simulink model "HevIpsPowertrainController"  (R2023b)
settings: configuration reference "VehicleFixed10ms" (kept outside this file)
undefined symbols (not defined in the file): CtrlBcuTrlrBrkGain, CtrlVcuHevIpsBattChrgPwrMax, CtrlVcuHevIpsBattDischrgPwrMax, CtrlVcuHevIpsChrgLmtBpt, CtrlVcuHevIpsDischrgLmtBpt, CtrlVcuHevIpsEngPwr, CtrlVcuHevIpsEngSpd, CtrlVcuHevIpsEngTrq, CtrlVcuHevIpsEngTrqWhl, CtrlVcuHevIpsEVSpdLmt, CtrlVcuHevIpsGenPwrMax, CtrlVcuHevIpsGenTrqMax, CtrlVcuHevIpsMotPwr, CtrlVcuHevIpsN_idle, CtrlVcuHevIpsNsysWhl, CtrlVcuHevIpsRegenBrkCutOff, CtrlVcuHevIpsRegenBrkSpdBpt, CtrlVcuHevIpsSocBpt, CtrlVcuHevIpsSOCChrgFactor, CtrlVcuHevIpsSOCmin, CtrlVcuHevIpsSOCtarget, CtrlVcuHevIpsSysTrqWhl, PlntBrkActrBoreFrnt, PlntBrkFrntBias, PlntBrkKinFricCffFrnt, PlntBrkNumPadsFrnt, PlntBrkPadMeanRadiusFrnt, PlntBrkPrsFctr, PlntBrkRearBias, PlntDiffrntlRatio, PlntEM1EffTbl, PlntEM1Spd, PlntEM1Trq, PlntEM1TrqEff, PlntEM2EffTbl, PlntEM2Spd, PlntEM2Trq, PlntEM2TrqEff, PlntHevIpsP1SunRingRatio, PlntHevIpsP2GearRatio
libraries: simulink x19, autolibutils x4, slpidlib x1
(part 1 of 2)
settings Model: DataDictionary=VirtualVehicleTemplate.sldd  ModifiedByFormat=The MathWorks, Inc.  Creator=The MathWorks, Inc.  LastModifiedBy=The MathWorks, Inc.
settings ConfigSetRef: SourceName=VehicleFixed10ms

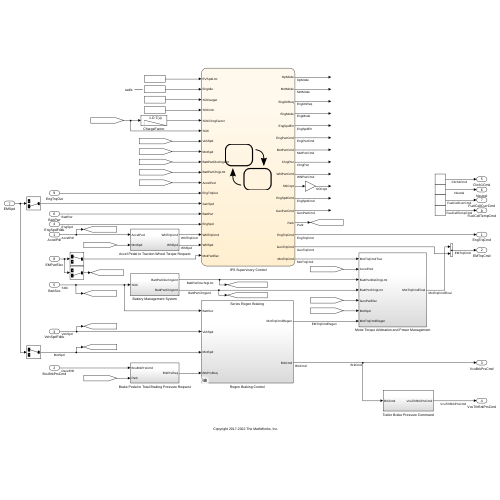
[thumbnail: Simulink's stored preview of the top-level diagram]
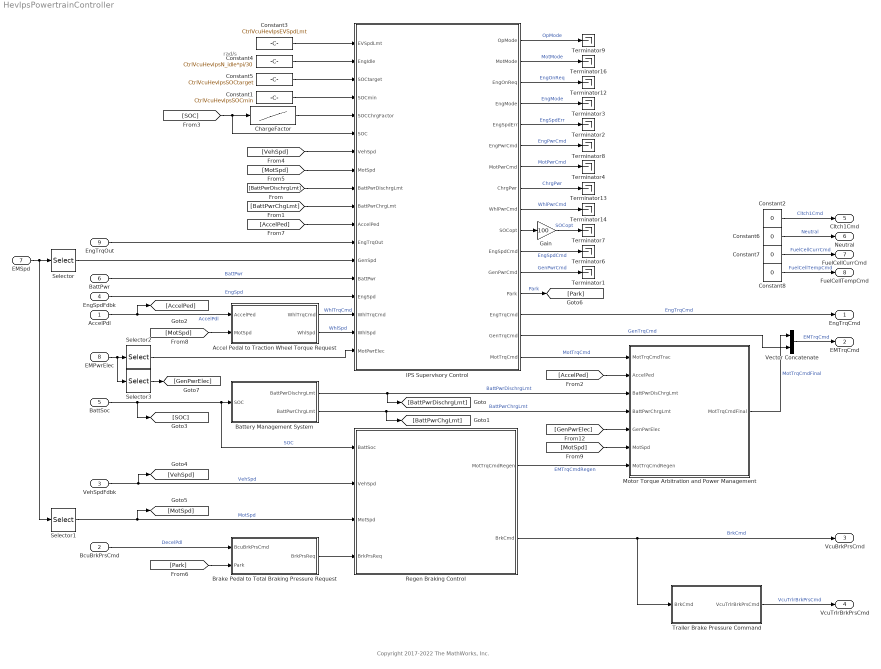
== system HevIpsPowertrainController ==
  note: rad/s
  note: Copyright 2017-2022 The MathWorks, Inc.
  AccelPdl : Inport  OutDataTypeStr=double  PortDimensions=1
  BcuBrkPrsCmd : Inport  Port=2  OutDataTypeStr=double  PortDimensions=4
  VehSpdFdbk : Inport  Port=3  OutDataTypeStr=double  PortDimensions=1
  EngSpdFdbk : Inport  Port=4  OutDataTypeStr=double  PortDimensions=1
  BattSoc : Inport  Port=5  OutDataTypeStr=double  PortDimensions=1
  BattPwr : Inport  Port=6  OutDataTypeStr=double  PortDimensions=1
  EMSpd : Inport  Port=7  OutDataTypeStr=double  PortDimensions=2
  EMPwrElec : Inport  Port=8  OutDataTypeStr=double  PortDimensions=2
  EngTrqOut : Inport  Port=9  OutDataTypeStr=double  PortDimensions=1
  Accel Pedal to Traction Wheel Torque Request : Subsystem  InitFcn=[~]=autosharedicon('autolibinternalvvblock',gcb,0);
  Battery Management System : Subsystem
  Brake Pedal to Total Braking Pressure Request : Subsystem
  ChargeFactor : Lookup_n-D  NumberOfTableDimensions=1  BreakpointsForDimension1=[20 80]  Table=CtrlVcuHevIpsSOCChrgFactor  ExtrapMethod=Clip  UseLastTableValue=on  InternalRulePriority=Speed  RndMeth=Simplest
  Constant1 : Constant  Value=CtrlVcuHevIpsSOCmin  SampleTime=-1
  Constant{2,6..8} (4 alike) : Constant  Value=0  SampleTime=-1
  Constant3 : Constant  Value=CtrlVcuHevIpsEVSpdLmt  SampleTime=-1
  Constant4 : Constant  Value=CtrlVcuHevIpsN_idle*pi/30  SampleTime=-1
  Constant5 : Constant  Value=CtrlVcuHevIpsSOCtarget  SampleTime=-1
  Gain : Gain  Gain=100
  IPS Supervisory Control : Stateflow chart  TreatAsAtomicUnit=on
  Motor Torque Arbitration and Power Management : Subsystem
  Regen Braking Control : Subsystem  Variant=on  VariantControlMode=label  VariantControl=(default)  LabelModeActiveChoice=Variant
  Selector : Selector  InputPortWidth=2  IndexOptions=Index vector (dialog)  Indices=[2]  OutputSizes=1
  Selector1 : Selector  InputPortWidth=2  IndexOptions=Index vector (dialog)  Indices=[1]  OutputSizes=1
  Selector2 : Selector  InputPortWidth=2  IndexOptions=Index vector (dialog)  Indices=[1]  OutputSizes=1
  Selector3 : Selector  InputPortWidth=2  IndexOptions=Index vector (dialog)  Indices=[2]  OutputSizes=1
  Terminator{1..4,6..9,12..14,16} (12 alike) : Terminator
  Trailer Brake Pressure Command : Subsystem
  Vector Concatenate : Concatenate
  EngTrqCmd : Outport  OutDataTypeStr=double  PortDimensions=1  VectorParamsAs1DForOutWhenUnconnected=off
  EMTrqCmd : Outport  Port=2  OutDataTypeStr=double  PortDimensions=2  VectorParamsAs1DForOutWhenUnconnected=off
  VcuBrkPrsCmd : Outport  Port=3  OutDataTypeStr=double  PortDimensions=4  VectorParamsAs1DForOutWhenUnconnected=off
  VcuTrlrBrkPrsCmd : Outport  Port=4  PortDimensions=6  VectorParamsAs1DForOutWhenUnconnected=off
  Cltch1Cmd : Outport  Port=5  OutDataTypeStr=double  PortDimensions=1  VectorParamsAs1DForOutWhenUnconnected=off
  Neutral : Outport  Port=6  OutDataTypeStr=double  PortDimensions=1  VectorParamsAs1DForOutWhenUnconnected=off
  FuelCellCurrCmd : Outport  Port=7  OutDataTypeStr=double  PortDimensions=1
  FuelCellTempCmd : Outport  Port=8  OutDataTypeStr=double  PortDimensions=1
  wires:
  AccelPdl/1 -> Accel Pedal to Traction Wheel Torque Request/1(AccelPed), [AccelPed]  "AccelPdl"
  BcuBrkPrsCmd/1 -> Brake Pedal to Total Braking Pressure Request/1(BcuBrkPrsCmd)  "DecelPdl"
  VehSpdFdbk/1 -> [VehSpd], Regen Braking Control/2("VehSpd ")  "VehSpd"
  EngSpdFdbk/1 -> IPS Supervisory Control/15(EngSpd)  "EngSpd"
  BattPwr/1 -> IPS Supervisory Control/14(BattPwr)  "BattPwr"
  BattSoc/1 -> [SOC], Regen Braking Control/1("BattSoc "), Battery Management System/1(SOC)  "SOC"
  Selector1/1 -> [MotSpd], Regen Braking Control/3("MotSpd ")  "MotSpd"
  Battery Management System/2(BattPwrChrgLmt) -> [BattPwrChgLmt], Motor Torque Arbitration and Power Management/4("BattPwrChrgLmt ")  "BattPwrChrgLmt"
  Battery Management System/1(BattPwrDischrgLmt) -> Motor Torque Arbitration and Power Management/3(BattPwrDisChrgLmt), [BattPwrDischrgLmt]  "BattPwrDischrgLmt"
  IPS Supervisory Control/1(OpMode) -> Terminator9/1  "OpMode"
  IPS Supervisory Control/6(EngPwrCmd) -> Terminator8/1  "EngPwrCmd"
  IPS Supervisory Control/3(EngOnReq) -> Terminator12/1  "EngOnReq"
  IPS Supervisory Control/7(MotPwrCmd) -> Terminator4/1  "MotPwrCmd"
  [SOC] -> IPS Supervisory Control/6(SOC), ChargeFactor/1
  [VehSpd] -> IPS Supervisory Control/7(VehSpd)
  Constant3/1 -> IPS Supervisory Control/1(EVSpdLmt)
  [BattPwrDischrgLmt] -> IPS Supervisory Control/9(BattPwrDischrgLmt)
  [BattPwrChgLmt] -> IPS Supervisory Control/10(BattPwrChrgLmt)
  Accel Pedal to Traction Wheel Torque Request/1(WhlTrqCmd) -> IPS Supervisory Control/16(WhlTrqCmd)  "WhlTrqCmd"
  Constant4/1 -> IPS Supervisory Control/2(EngIdle)
  Accel Pedal to Traction Wheel Torque Request/2(WhlSpd) -> IPS Supervisory Control/17(WhlSpd)  "WhlSpd"
  IPS Supervisory Control/16(MotTrqCmd) -> Motor Torque Arbitration and Power Management/1(MotTrqCmdTrac)  "MotTrqCmd"
  Brake Pedal to Total Braking Pressure Request/1(BrkPrsReq) -> Regen Braking Control/4("BrkPrsReq ")
  Regen Braking Control/1(" MotTrqCmdRegen") -> Motor Torque Arbitration and Power Management/7(MotTrqCmdRegen)  "EMTrqCmdRegen"
  IPS Supervisory Control/10(SOCopt) -> Gain/1
  IPS Supervisory Control/8(ChrgPwr) -> Terminator13/1  "ChrgPwr"
  IPS Supervisory Control/9(WhlPwrCmd) -> Terminator14/1  "WhlPwrCmd"
  [MotSpd] -> IPS Supervisory Control/8(MotSpd)
  Gain/1 -> Terminator7/1  "SOCopt"
  IPS Supervisory Control/4(EngMode) -> Terminator3/1  "EngMode"
  IPS Supervisory Control/11(EngSpdCmd) -> Terminator6/1  "EngSpdCmd"
  IPS Supervisory Control/2(MotMode) -> Terminator16/1  "MotMode"
  Constant5/1 -> IPS Supervisory Control/3(SOCtarget)
  ChargeFactor/1 -> IPS Supervisory Control/5(SOCChrgFactor)
  [AccelPed] -> IPS Supervisory Control/11(AccelPed)
  IPS Supervisory Control/5(EngSpdErr) -> Terminator2/1  "EngSpdErr"
  [MotSpd] -> Accel Pedal to Traction Wheel Torque Request/2(MotSpd)
  [AccelPed] -> Motor Torque Arbitration and Power Management/2(AccelPed)
  Selector/1 -> IPS Supervisory Control/13(GenSpd)
  Selector3/1 -> [GenPwrElec]
  IPS Supervisory Control/12(GenPwrCmd) -> Terminator1/1  "GenPwrCmd"
  EMPwrElec/1 -> Selector3/1, Selector2/1
  Motor Torque Arbitration and Power Management/1(MotTrqCmdFinal) -> Vector Concatenate/1  "MotTrqCmdFinal"
  Constant1/1 -> IPS Supervisory Control/4(SOCmin)
  IPS Supervisory Control/15(GenTrqCmd) -> Vector Concatenate/2  "GenTrqCmd"
  IPS Supervisory Control/14(EngTrqCmd) -> EngTrqCmd/1  "EngTrqCmd"
  EngTrqOut/1 -> IPS Supervisory Control/12(EngTrqOut)
  IPS Supervisory Control/13(Park) -> [Park]  "Park"
  [Park] -> Brake Pedal to Total Braking Pressure Request/2(Park)
  [MotSpd] -> Motor Torque Arbitration and Power Management/6(MotSpd)
  [GenPwrElec] -> Motor Torque Arbitration and Power Management/5(GenPwrElec)
  Vector Concatenate/1 -> EMTrqCmd/1  "EMTrqCmd"
  EMSpd/1 -> Selector1/1, Selector/1
  Constant6/1 -> Neutral/1  "Neutral"
  Constant2/1 -> Cltch1Cmd/1  "Cltch1Cmd"
  Selector2/1 -> IPS Supervisory Control/18(MotPwrElec)
  Constant7/1 -> FuelCellCurrCmd/1  "FuelCellCurrCmd"
  Constant8/1 -> FuelCellTempCmd/1  "FuelCellTempCmd"
  Regen Braking Control/2(" BrkCmd") -> Trailer Brake Pressure Command/1(BrkCmd), VcuBrkPrsCmd/1  "BrkCmd"
  Trailer Brake Pressure Command/1(VcuTrlrBrkPrsCmd) -> VcuTrlrBrkPrsCmd/1  "VcuTrlrBrkPrsCmd"

== system HevIpsPowertrainController/Accel Pedal to Traction Wheel Torque Request ==
  AccelPed : Inport
  MotSpd : Inport  Port=2
  MaxSysTrqWhlVsWhlSpd : Lookup_n-D  NumberOfTableDimensions=1  BreakpointsForDimension1=CtrlVcuHevIpsNsysWhl  Table=CtrlVcuHevIpsSysTrqWhl  ExtrapMethod=Clip  UseLastTableValue=on  InternalRulePriority=Speed  OutDataTypeStr=Inherit: Inherit from 'Table data'  RndMeth=Simplest
  MotSpdToWhlSpd : Gain  Gain=1/(PlntHevIpsP2GearRatio)/PlntDiffrntlRatio
  Product1 : Product
  rads_to_rpm : Gain  Gain=30/pi
  WhlTrqCmd : Outport  VectorParamsAs1DForOutWhenUnconnected=off
  WhlSpd : Outport  Port=2  VectorParamsAs1DForOutWhenUnconnected=off
  wires:
  rads_to_rpm/1 -> MaxSysTrqWhlVsWhlSpd/1
  MotSpdToWhlSpd/1 -> rads_to_rpm/1, WhlSpd/1
  Product1/1 -> WhlTrqCmd/1
  MotSpd/1 -> MotSpdToWhlSpd/1
  MaxSysTrqWhlVsWhlSpd/1 -> Product1/2
  AccelPed/1 -> Product1/1

== system HevIpsPowertrainController/Battery Management System ==
  note: Limit battery charge / discharge power based on SOC
  SOC : Inport
  ChrgLmt : Lookup_n-D  NumberOfTableDimensions=1  BreakpointsForDimension1=CtrlVcuHevIpsSocBpt  Table=CtrlVcuHevIpsChrgLmtBpt  ExtrapMethod=Clip  UseLastTableValue=on  InternalRulePriority=Speed  RndMeth=Simplest
  DischrgLmt : Lookup_n-D  NumberOfTableDimensions=1  BreakpointsForDimension1=CtrlVcuHevIpsSocBpt  Table=CtrlVcuHevIpsDischrgLmtBpt  ExtrapMethod=Clip  UseLastTableValue=on  InternalRulePriority=Speed  RndMeth=Simplest
  MaxChrg : Constant  Value=CtrlVcuHevIpsBattChrgPwrMax  SampleTime=-1
  MaxDischrg : Constant  Value=CtrlVcuHevIpsBattDischrgPwrMax  SampleTime=-1
  Product : Product
  Product1 : Product
  BattPwrDischrgLmt : Outport  VectorParamsAs1DForOutWhenUnconnected=off
  BattPwrChrgLmt : Outport  Port=2  VectorParamsAs1DForOutWhenUnconnected=off
  wires:
  SOC/1 -> DischrgLmt/1, ChrgLmt/1
  MaxChrg/1 -> Product1/2
  MaxDischrg/1 -> Product/2
  Product/1 -> BattPwrDischrgLmt/1
  Product1/1 -> BattPwrChrgLmt/1
  ChrgLmt/1 -> Product1/1
  DischrgLmt/1 -> Product/1

== system HevIpsPowertrainController/Brake Pedal to Total Braking Pressure Request ==
  BcuBrkPrsCmd : Inport
  Park : Inport  Port=2
  Front Bias : Constant  Value=PlntBrkFrntBias
  Gain4 : Gain  Gain=PlntBrkPrsFctr
  Mux : Mux
  Product : Product
  Rear Bias : Constant  Value=PlntBrkRearBias
  Terminator : Terminator
  BrkPrsReq : Outport  VectorParamsAs1DForOutWhenUnconnected=off
  wires:
  BcuBrkPrsCmd/1 -> Product/2
  Mux/1 -> Product/1
  Rear Bias/1 -> Mux/4, Mux/3
  Front Bias/1 -> Mux/1, Mux/2
  Gain4/1 -> BrkPrsReq/1
  Product/1 -> Gain4/1
  Park/1 -> Terminator/1

== system HevIpsPowertrainController/IPS Supervisory Control/Engine_Control.Run.TrqCalc ==
  EngPwrCmd : Inport
  f : TriggerPort  TriggerType=function-call  VariantControl=Variant  StatesWhenEnabling=reset
      settings: CopyFcn=Stateflow.SLINSF.SimulinkMan.removeBlockPreDeleteFcn  PreDeleteFcn=Stateflow.SLINSF.SimulinkMan.unsafePredeleteFcn
  OptimalEngineSpeed : Lookup_n-D  NumberOfTableDimensions=1  BreakpointsForDimension1=[0 CtrlVcuHevIpsEngPwr(1,1:15)]  Table=[CtrlVcuHevIpsN_idle CtrlVcuHevIpsEngSpd(1,1:15)]  ExtrapMethod=Clip  UseLastTableValue=on  InternalRulePriority=Speed  RndMeth=Simplest
  OptimalEngineTorque : Lookup_n-D  NumberOfTableDimensions=1  BreakpointsForDimension1=[0 CtrlVcuHevIpsEngPwr(1,1:15)]  Table=[0 CtrlVcuHevIpsEngTrq(1,1:15)]  ExtrapMethod=Clip  UseLastTableValue=on  InternalRulePriority=Speed  RndMeth=Simplest
  rpm_to_rads : Gain  Gain=pi/30
  EngTrqCmd : Outport  VectorParamsAs1DForOutWhenUnconnected=off
  EngSpdCmd : Outport  Port=2  VectorParamsAs1DForOutWhenUnconnected=off
  wires:
  rpm_to_rads/1 -> EngSpdCmd/1
  OptimalEngineSpeed/1 -> rpm_to_rads/1
  EngPwrCmd/1 -> OptimalEngineTorque/1, OptimalEngineSpeed/1
  OptimalEngineTorque/1 -> EngTrqCmd/1

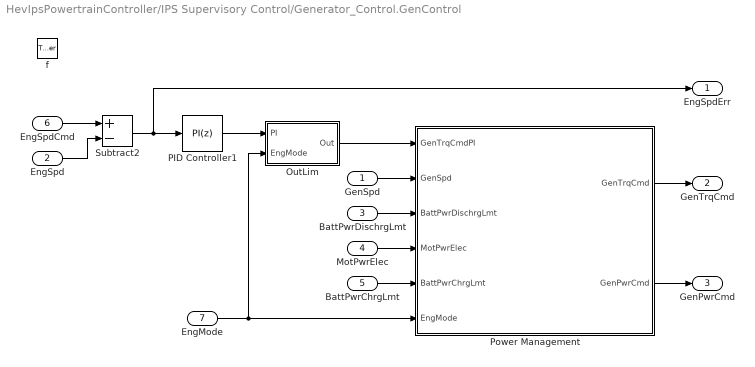
== system HevIpsPowertrainController/IPS Supervisory Control/Generator_Control.GenControl ==
  GenSpd : Inport
  EngSpd : Inport  Port=2
  BattPwrDischrgLmt : Inport  Port=3
  MotPwrElec : Inport  Port=4
  BattPwrChrgLmt : Inport  Port=5
  EngSpdCmd : Inport  Port=6
  EngMode : Inport  Port=7
  f : TriggerPort  TriggerType=function-call  VariantControl=Variant  StatesWhenEnabling=reset  SampleTime=-1
      settings: CopyFcn=Stateflow.SLINSF.SimulinkMan.removeBlockPreDeleteFcn  PreDeleteFcn=Stateflow.SLINSF.SimulinkMan.unsafePredeleteFcn
  OutLim : Subsystem
  PID Controller1 : slpidlib/PID Controller  Controller=PI  Form=Parallel  TimeDomain=Discrete-time  UseExternalTs=off  SampleTime=-1  IntegratorMethod=Forward Euler  FilterMethod=Forward Euler  ControllerParametersSource=internal  P=1  I=0.5  UseKiTs=off  D=1  N=100  UseFilter=on  TunerSelectOption=Transfer Function Based (PID Tuner App)  ZeroCross=off  InitialConditionSource=internal  InitialConditionForIntegrator=0  InitialConditionForFilter=0  DifferentiatorICPrevScaledInput=0  ExternalReset=none  TrackingMode=off  Kt=1  LimitOutput=on  SatLimitsSource=internal  UpperSaturationLimit=CtrlVcuHevIpsGenTrqMax  LowerSaturationLimit=-CtrlVcuHevIpsGenTrqMax  LinearizeAsGain=on  AntiWindupMode=clamping  Kb=1  LimitIntegrator=off  UpperIntegratorSaturationLimit=inf  LowerIntegratorSaturationLimit=-inf  POutMin=[]  POutMax=[]  IOutMin=[]  IOutMax=[]  DOutMin=[]  DOutMax=[]  NOutMin=[]  NOutMax=[]  SumOutMin=[]  SumOutMax=[]  SaturationOutMin=[]  SaturationOutMax=[]  PParamMin=[]  PParamMax=[]  IParamMin=[]  IParamMax=[]  DParamMin=[]  DParamMax=[]  NParamMin=[]  NParamMax=[]  KbParamMin=[]  KbParamMax=[]  KtParamMin=[]  KtParamMax=[]  KbOutMin=[]  KbOutMax=[]  KtOutMin=[]  KtOutMax=[]  IntegratorOutMin=[]  IntegratorOutMax=[]  FilterOutMin=[]  FilterOutMax=[]  SumI1OutMin=[]  SumI1OutMax=[]  SumI2OutMin=[]  SumI2OutMax=[]  SumI3OutMin=[]  SumI3OutMax=[]  SumI4OutMin=[]  SumI4OutMax=[]  SumDOutMin=[]  SumDOutMax=[]  DifferentiatorOutMin=[]  DifferentiatorOutMax=[]  FilterDiffOutCoefMin=[]  FilterDiffOutCoefMax=[]  ReciprocalOutMin=[]  ReciprocalOutMax=[]  SumDenOutMin=[]  SumDenOutMax=[]  SumNumOutMin=[]  SumNumOutMax=[]  DivideOutMin=[]  DivideOutMax=[]  UdiffTsProdOutMin=[]  UdiffTsProdOutMax=[]  NTsProdOutMin=[]  NTsProdOutMax=[]  UintegralTsProdOutMin=[]  UintegralTsProdOutMax=[]  UngainTsProdOutMin=[]  UngainTsProdOutMax=[]  ClampingZeroOutDataTypeStr=Inherit: Inherit via back propagation  ClampingZeroOutMin=[]  ClampingZeroOutMax=[]  FilterDenConstantOutDataTypeStr=Inherit: Inherit via back propagation  FilterDenConstantOutMin=[]  FilterDenConstantOutMax=[]  PCopyOutDataTypeStr=Inherit: Inherit via back propagation  PCopyOutMin=[]  PCopyOutMax=[]  NCopyOutDataTypeStr=Inherit: Inherit via back propagation  NCopyOutMin=[]  NCopyOutMax=[]  IntegratorContinuousStateAttributes=''  IntegratorStateMustResolveToSignalObject=off  IntegratorRTWStateStorageClass=Auto  FilterContinuousStateAttributes=''  FilterStateMustResolveToSignalObject=off  FilterRTWStateStorageClass=Auto  ParallelPVariant=InternalParameters  IdealPVariant=Disabled  IVariant=InternalParameters  DVariant=Disabled  IntegratorVariant=Discrete  SatVariant=Enabled  AWVariant=DiscClampingParallel  PCopyVariant=Disabled  TRVariant=Disabled  FdbkBlocksVariant=Forward  IdealPFdbkVariant=Disabled  SatFdbkVariant=Disabled  DerivativeFilterVariant=Disabled  NVariant=Disabled  NCopyVariant=Disabled_SignalSpec  FilterICVariant=Disabled  IntegratorICVariant=InternalICs  ExternalResetVariant=Disabled  TRSumVariant=Passthrough  SumFdbkVariant=Disabled  SumVariant=Sum_PI  TsampFilterVariant=InternalTs  TsampNgainVariant=Passthrough  TsampIntegralVariant=Disabled_SignalSpec  ExternalSaturationOutDataTypeStr=Inherit: Same as second input
  Power Management : Subsystem
  Subtract2 : Sum  Inputs=+-
  EngSpdErr : Outport  VectorParamsAs1DForOutWhenUnconnected=off
  GenTrqCmd : Outport  Port=2  VectorParamsAs1DForOutWhenUnconnected=off
  GenPwrCmd : Outport  Port=3  VectorParamsAs1DForOutWhenUnconnected=off
  wires:
  Subtract2/1 -> PID Controller1/1, EngSpdErr/1
  EngSpd/1 -> Subtract2/2
  MotPwrElec/1 -> Power Management/4(MotPwrElec)
  BattPwrDischrgLmt/1 -> Power Management/3(BattPwrDischrgLmt)
  BattPwrChrgLmt/1 -> Power Management/5(BattPwrChrgLmt)
  GenSpd/1 -> Power Management/2(GenSpd)
  EngSpdCmd/1 -> Subtract2/1
  EngMode/1 -> OutLim/2(EngMode), Power Management/6(EngMode)
  Power Management/1(GenTrqCmd) -> GenTrqCmd/1
  Power Management/2(GenPwrCmd) -> GenPwrCmd/1
  PID Controller1/1 -> OutLim/1(PI)
  OutLim/1(Out) -> Power Management/1(GenTrqCmdPI)

== system HevIpsPowertrainController/IPS Supervisory Control/Motor_Control.Mot_EV.MotTrqEV ==
  WhlTrqCmd : Inport
  f : TriggerPort  TriggerType=function-call  VariantControl=Variant  StatesWhenEnabling=reset
      settings: CopyFcn=Stateflow.SLINSF.SimulinkMan.removeBlockPreDeleteFcn  PreDeleteFcn=Stateflow.SLINSF.SimulinkMan.unsafePredeleteFcn
  WhlTrqReflectedMotTrq : Gain  Gain=1/(PlntHevIpsP2GearRatio)/PlntDiffrntlRatio
  MotTrqCmd : Outport  VectorParamsAs1DForOutWhenUnconnected=off
  wires:
  WhlTrqCmd/1 -> WhlTrqReflectedMotTrq/1
  WhlTrqReflectedMotTrq/1 -> MotTrqCmd/1

== system HevIpsPowertrainController/IPS Supervisory Control/Motor_Control.Mot_HEV.MotTrqHEV ==
  MotPwrCmd : Inport
  MotSpd : Inport  Port=2
  f : TriggerPort  TriggerType=function-call  VariantControl=Variant  StatesWhenEnabling=reset
      settings: CopyFcn=Stateflow.SLINSF.SimulinkMan.removeBlockPreDeleteFcn  PreDeleteFcn=Stateflow.SLINSF.SimulinkMan.unsafePredeleteFcn
  Elec_to_MechPwr1 : Product  Inputs=*/
  div0protect - poly1 : autolibutils/div0protect - poly  thresh=2  ZeroCross1=off  aMode=aMode
  MotTrqCmd : Outport  VectorParamsAs1DForOutWhenUnconnected=off
  wires:
  MotPwrCmd/1 -> Elec_to_MechPwr1/1
  MotSpd/1 -> div0protect - poly1/1
  div0protect - poly1/1 -> Elec_to_MechPwr1/2
  Elec_to_MechPwr1/1 -> MotTrqCmd/1

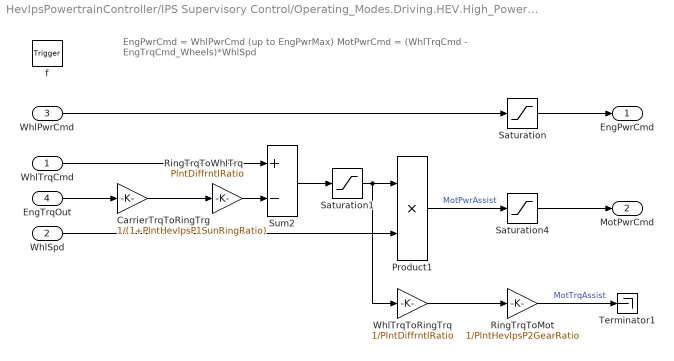
== system HevIpsPowertrainController/IPS Supervisory Control/Operating_Modes.Driving.HEV.High_Power_Charge_Deplete.OpMode4 ==
  note: EngPwrCmd = WhlPwrCmd (up to EngPwrMax)
      | MotPwrCmd =  (WhlTrqCmd - EngTrqCmd_Wheels)*WhlSpd
  WhlTrqCmd : Inport
  WhlSpd : Inport  Port=2
  WhlPwrCmd : Inport  Port=3
  EngTrqOut : Inport  Port=4
  f : TriggerPort  TriggerType=function-call  VariantControl=Variant  StatesWhenEnabling=reset
      settings: CopyFcn=Stateflow.SLINSF.SimulinkMan.removeBlockPreDeleteFcn  PreDeleteFcn=Stateflow.SLINSF.SimulinkMan.unsafePredeleteFcn
  CarrierTrqToRingTrg : Gain  Gain=1/(1+PlntHevIpsP1SunRingRatio)
  Product1 : Product
  RingTrqToMot : Gain  Gain=1/PlntHevIpsP2GearRatio
  RingTrqToWhlTrq : Gain  Gain=PlntDiffrntlRatio
  Saturation : Saturate  UpperLimit=max(CtrlVcuHevIpsEngPwr(1,1:15))  LowerLimit=0
  Saturation1 : Saturate  UpperLimit=inf  LowerLimit=0
  Saturation4 : Saturate  UpperLimit=max(CtrlVcuHevIpsMotPwr)  LowerLimit=0
  Sum2 : Sum  Inputs=+-
  Terminator1 : Terminator
  WhlTrqToRingTrq : Gain  Gain=1/PlntDiffrntlRatio
  EngPwrCmd : Outport  VectorParamsAs1DForOutWhenUnconnected=off
  MotPwrCmd : Outport  Port=2  VectorParamsAs1DForOutWhenUnconnected=off
  wires:
  CarrierTrqToRingTrg/1 -> RingTrqToWhlTrq/1
  WhlSpd/1 -> Product1/2
  WhlTrqCmd/1 -> Sum2/1
  RingTrqToWhlTrq/1 -> Sum2/2
  Sum2/1 -> Saturation1/1
  Saturation1/1 -> WhlTrqToRingTrq/1, Product1/1
  WhlTrqToRingTrq/1 -> RingTrqToMot/1
  RingTrqToMot/1 -> Terminator1/1  "MotTrqAssist"
  Product1/1 -> Saturation4/1  "MotPwrAssist"
  EngTrqOut/1 -> CarrierTrqToRingTrg/1
  Saturation/1 -> EngPwrCmd/1
  WhlPwrCmd/1 -> Saturation/1
  Saturation4/1 -> MotPwrCmd/1

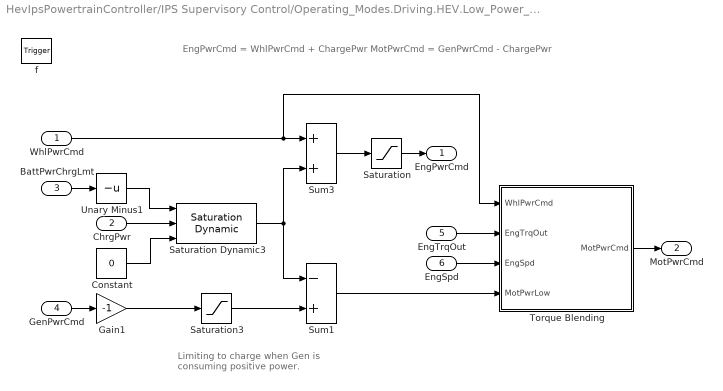
== system HevIpsPowertrainController/IPS Supervisory Control/Operating_Modes.Driving.HEV.Low_Power_Charge_Sustain.OpMode3 ==
  note: Limiting to charge when Gen
      | is consuming positive power.
  note: EngPwrCmd = WhlPwrCmd + ChargePwr
      | MotPwrCmd = GenPwrCmd - ChargePwr
  WhlPwrCmd : Inport
  ChrgPwr : Inport  Port=2
  BattPwrChrgLmt : Inport  Port=3
  GenPwrCmd : Inport  Port=4
  EngTrqOut : Inport  Port=5
  EngSpd : Inport  Port=6
  f : TriggerPort  TriggerType=function-call  VariantControl=Variant  StatesWhenEnabling=reset
      settings: CopyFcn=Stateflow.SLINSF.SimulinkMan.removeBlockPreDeleteFcn  PreDeleteFcn=Stateflow.SLINSF.SimulinkMan.unsafePredeleteFcn
  Constant : Constant  Value=0
  Gain1 : Gain  Gain=-1
  Saturation : Saturate  UpperLimit=max(CtrlVcuHevIpsEngPwr(1,1:15))  LowerLimit=0
  Saturation Dynamic3 : simulink/Discontinuities/Saturation Dynamic  OutMin=[]  OutMax=[]  OutDataTypeStr=Inherit: Same as second input  OutDataType=fixdt(1, 16)  OutScaling=2^-10  DoSatur=off
  Saturation3 : Saturate  UpperLimit=0  LowerLimit=-CtrlVcuHevIpsGenPwrMax
  Sum1 : Sum  Inputs=-+
  Sum3 : Sum
  Torque Blending : Subsystem
  Unary Minus1 : UnaryMinus
  EngPwrCmd : Outport  VectorParamsAs1DForOutWhenUnconnected=off
  MotPwrCmd : Outport  Port=2  VectorParamsAs1DForOutWhenUnconnected=off
  wires:
  Unary Minus1/1 -> Saturation Dynamic3/1
  Sum3/1 -> Saturation/1
  ChrgPwr/1 -> Saturation Dynamic3/2
  Saturation/1 -> EngPwrCmd/1
  Saturation Dynamic3/1 -> Sum1/1, Sum3/2
  GenPwrCmd/1 -> Gain1/1
  Gain1/1 -> Saturation3/1
  BattPwrChrgLmt/1 -> Unary Minus1/1
  Constant/1 -> Saturation Dynamic3/3
  WhlPwrCmd/1 -> Sum3/1, Torque Blending/1(WhlPwrCmd)
  Saturation3/1 -> Sum1/2
  EngTrqOut/1 -> Torque Blending/2(EngTrqOut)
  EngSpd/1 -> Torque Blending/3(EngSpd)
  Sum1/1 -> Torque Blending/4(MotPwrLow)
  Torque Blending/1(MotPwrCmd) -> MotPwrCmd/1

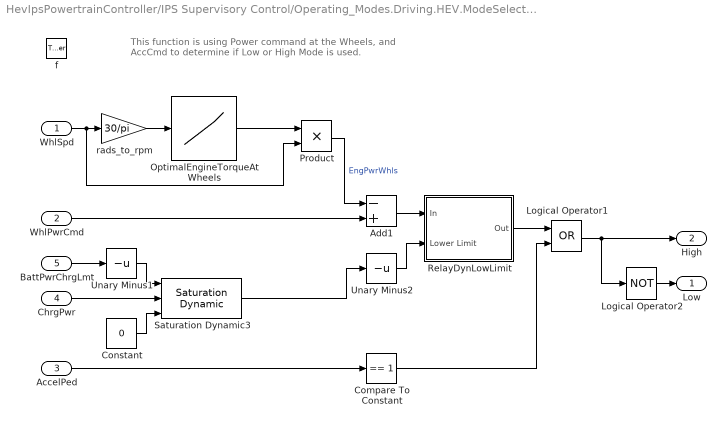
== system HevIpsPowertrainController/IPS Supervisory Control/Operating_Modes.Driving.HEV.ModeSelection ==
  note: This function is using Power command at the Wheels,
      | and AccCmd to determine if Low or High Mode is used.
  WhlSpd : Inport  PortDimensions=1
  WhlPwrCmd : Inport  Port=2  PortDimensions=1
  AccelPed : Inport  Port=3  PortDimensions=1
  ChrgPwr : Inport  Port=4
  BattPwrChrgLmt : Inport  Port=5
  f : TriggerPort  TriggerType=function-call  VariantControl=Variant  StatesWhenEnabling=reset
      settings: CopyFcn=Stateflow.SLINSF.SimulinkMan.removeBlockPreDeleteFcn  PreDeleteFcn=Stateflow.SLINSF.SimulinkMan.unsafePredeleteFcn
  Add1 : Sum  Inputs=-+
  Compare To Constant : simulink/Logic and Bit Operations/Compare To Constant  relop===  const=1  OutDataTypeStr=boolean
  Constant : Constant  Value=0
  Logical Operator1 : Logic  Operator=OR  AllPortsSameDT=off  OutDataTypeStr=boolean
  Logical Operator2 : Logic  Operator=NOT  AllPortsSameDT=off  OutDataTypeStr=boolean
  OptimalEngineTorqueAtWheels : Lookup_n-D  NumberOfTableDimensions=1  BreakpointsForDimension1=CtrlVcuHevIpsNsysWhl  Table=CtrlVcuHevIpsEngTrqWhl  ExtrapMethod=Clip  UseLastTableValue=on  InternalRulePriority=Speed  RndMeth=Simplest
  Product : Product
  RelayDynLowLimit : Subsystem
  Saturation Dynamic3 : simulink/Discontinuities/Saturation Dynamic  OutMin=[]  OutMax=[]  OutDataTypeStr=Inherit: Same as second input  OutDataType=fixdt(1, 16)  OutScaling=2^-10  DoSatur=off
  Unary Minus1 : UnaryMinus
  Unary Minus2 : UnaryMinus
  rads_to_rpm : Gain  Gain=30/pi
  Low : Outport  VectorParamsAs1DForOutWhenUnconnected=off
  High : Outport  Port=2  VectorParamsAs1DForOutWhenUnconnected=off
  wires:
  WhlSpd/1 -> Product/2, rads_to_rpm/1
  rads_to_rpm/1 -> OptimalEngineTorqueAtWheels/1
  OptimalEngineTorqueAtWheels/1 -> Product/1
  Compare To Constant/1 -> Logical Operator1/2
  Logical Operator1/1 -> Logical Operator2/1, High/1
  Product/1 -> Add1/1  "EngPwrWhls"
  Constant/1 -> Saturation Dynamic3/3
  BattPwrChrgLmt/1 -> Unary Minus1/1
  ChrgPwr/1 -> Saturation Dynamic3/2
  Unary Minus1/1 -> Saturation Dynamic3/1
  Saturation Dynamic3/1 -> Unary Minus2/1
  WhlPwrCmd/1 -> Add1/2
  Logical Operator2/1 -> Low/1
  RelayDynLowLimit/1(Out) -> Logical Operator1/1
  Add1/1 -> RelayDynLowLimit/1(In)
  Unary Minus2/1 -> RelayDynLowLimit/2(Lower Limit)
  AccelPed/1 -> Compare To Constant/1

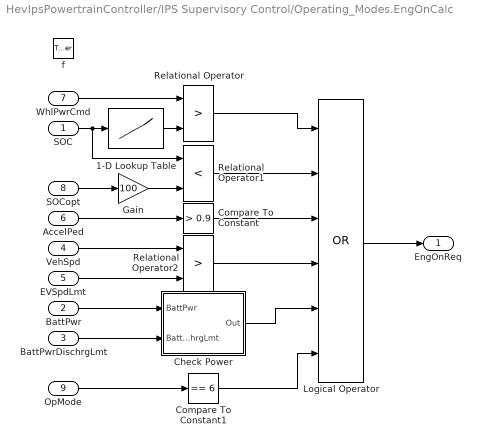
== system HevIpsPowertrainController/IPS Supervisory Control/Operating_Modes.EngOnCalc ==
  SOC : Inport
  BattPwr : Inport  Port=2
  BattPwrDischrgLmt : Inport  Port=3
  VehSpd : Inport  Port=4
  EVSpdLmt : Inport  Port=5
  AccelPed : Inport  Port=6
  WhlPwrCmd : Inport  Port=7
  SOCopt : Inport  Port=8
  OpMode : Inport  Port=9
  f : TriggerPort  TriggerType=function-call  VariantControl=Variant  StatesWhenEnabling=reset
      settings: CopyFcn=Stateflow.SLINSF.SimulinkMan.removeBlockPreDeleteFcn  PreDeleteFcn=Stateflow.SLINSF.SimulinkMan.unsafePredeleteFcn
  1-D Lookup Table : Lookup_n-D  NumberOfTableDimensions=1  BreakpointsForDimension1=[55 70]  Table=[CtrlVcuHevIpsEngPwr(1) CtrlVcuHevIpsEngPwr(2)]  ExtrapMethod=Clip  UseLastTableValue=on  InternalRulePriority=Speed  RndMeth=Simplest
  Check Power : Subsystem
  Compare To Constant : simulink/Logic and Bit Operations/Compare To Constant  relop=>  const=0.9  OutDataTypeStr=boolean
  Compare To Constant1 : simulink/Logic and Bit Operations/Compare To Constant  relop===  const=6  OutDataTypeStr=boolean
  Gain : Gain  Gain=100
  Logical Operator : Logic  Operator=OR  Inputs=6  AllPortsSameDT=off  OutDataTypeStr=boolean
  Relational Operator : RelationalOperator  Operator=>  OutDataTypeStr=boolean  RndMeth=Simplest  InputSameDT=off
  Relational Operator1 : RelationalOperator  Operator=<  OutDataTypeStr=boolean  RndMeth=Simplest  InputSameDT=off
  Relational Operator2 : RelationalOperator  Operator=>  OutDataTypeStr=boolean  RndMeth=Simplest  InputSameDT=off
  EngOnReq : Outport  VectorParamsAs1DForOutWhenUnconnected=off
  wires:
  BattPwrDischrgLmt/1 -> Check Power/2(BattPwrDischrgLmt)
  BattPwr/1 -> Check Power/1(BattPwr)
  Logical Operator/1 -> EngOnReq/1
  Relational Operator2/1 -> Logical Operator/4
  EVSpdLmt/1 -> Relational Operator2/2
  VehSpd/1 -> Relational Operator2/1
  AccelPed/1 -> Compare To Constant/1
  Compare To Constant/1 -> Logical Operator/3
  Check Power/1(Out) -> Logical Operator/5
  SOC/1 -> Relational Operator1/1, 1-D Lookup Table/1
  Relational Operator/1 -> Logical Operator/1
  1-D Lookup Table/1 -> Relational Operator/2
  SOCopt/1 -> Gain/1
  OpMode/1 -> Compare To Constant1/1
  Compare To Constant1/1 -> Logical Operator/6
  Relational Operator1/1 -> Logical Operator/2
  WhlPwrCmd/1 -> Relational Operator/1
  Gain/1 -> Relational Operator1/2

== system HevIpsPowertrainController/IPS Supervisory Control/Operating_Modes.Stationary.Charging.ChargePowerCalc ==
  SOC : Inport
  f : TriggerPort  TriggerType=function-call  VariantControl=Variant  StatesWhenEnabling=reset
      settings: CopyFcn=Stateflow.SLINSF.SimulinkMan.removeBlockPreDeleteFcn  PreDeleteFcn=Stateflow.SLINSF.SimulinkMan.unsafePredeleteFcn
  Charge Power : Lookup_n-D  NumberOfTableDimensions=1  BreakpointsForDimension1=[20 CtrlVcuHevIpsSOCtarget]  Table=[20000 0]  ExtrapMethod=Clip  UseLastTableValue=on  InternalRulePriority=Speed  RndMeth=Simplest
  EngPwrCmd : Outport  VectorParamsAs1DForOutWhenUnconnected=off
  wires:
  SOC/1 -> Charge Power/1
  Charge Power/1 -> EngPwrCmd/1

== system HevIpsPowertrainController/Motor Torque Arbitration and Power Management ==
  MotTrqCmdTrac : Inport
  AccelPed : Inport  Port=2
  BattPwrDisChrgLmt : Inport  Port=3
  "BattPwrChrgLmt " : Inport  Port=4
  GenPwrElec : Inport  Port=5
  MotSpd : Inport  Port=6
  MotTrqCmdRegen : Inport  Port=7
  Accel Decel Switch : Switch  Criteria=u2 > Threshold  SaturateOnIntegerOverflow=off  InputSameDT=off
  Compare To Constant : simulink/Logic and Bit Operations/Compare To Constant  relop=>  const=0  OutDataTypeStr=boolean
  Power Management : Subsystem
  MotTrqCmdFinal : Outport  VectorParamsAs1DForOutWhenUnconnected=off
  wires:
  AccelPed/1 -> Compare To Constant/1
  MotTrqCmdRegen/1 -> Accel Decel Switch/3
  Compare To Constant/1 -> Accel Decel Switch/2
  MotTrqCmdTrac/1 -> Accel Decel Switch/1
  Power Management/1(MotTrqLim) -> MotTrqCmdFinal/1
  Accel Decel Switch/1 -> Power Management/5(MotTrqCmd)
  BattPwrDisChrgLmt/1 -> Power Management/1(BattPwrDischrgLmt)
  GenPwrElec/1 -> Power Management/2(GenPwrElec)
  "BattPwrChrgLmt "/1 -> Power Management/3(BattPwrChrgLmt)
  MotSpd/1 -> Power Management/4(MotSpd)

== system HevIpsPowertrainController/Regen Braking Control ==
  "BattSoc " : Inport
  "VehSpd " : Inport  Port=2
  "MotSpd " : Inport  Port=3
  "BrkPrsReq " : Inport  Port=4
  Parallel Regen Braking : Subsystem  InitFcn=[~]=autosharedicon('autolibinternalvvblock',gcb,0);  VariantControl=(default)
  Series Regen Braking : Subsystem  InitFcn=[~]=autosharedicon('autolibinternalvvblock',gcb,0);  VariantControl=Variant
  " MotTrqCmdRegen" : Outport  VectorParamsAs1DForOutWhenUnconnected=off
  " BrkCmd" : Outport  Port=2  VectorParamsAs1DForOutWhenUnconnected=off

== system HevIpsPowertrainController/Trailer Brake Pressure Command ==
  BrkCmd : Inport
  Gain1 : Gain  Gain=CtrlBcuTrlrBrkGain
  Probe : Probe  ProbeSampleTime=off  ProbeComplexSignal=off
  Product : Product  Inputs=*/
  Selector2 : Selector  InputPortWidth=1  IndexOptions=Index vector (dialog)  Indices=[1 1 1 1 1 1]  OutputSizes=1
  Sum : Sum  Inputs=+
  VcuTrlrBrkPrsCmd : Outport
  wires:
  Gain1/1 -> Selector2/1
  Product/1 -> Gain1/1
  Probe/1 -> Product/2
  BrkCmd/1 -> Probe/1, Sum/1
  Sum/1 -> Product/1
  Selector2/1 -> VcuTrlrBrkPrsCmd/1

== system HevIpsPowertrainController/IPS Supervisory Control/Generator_Control.GenControl/OutLim ==
  PI : Inport
  EngMode : Inport  Port=2
  Compare To Constant : simulink/Logic and Bit Operations/Compare To Constant  relop===  const=3  OutDataTypeStr=boolean
  Constant : Constant  Value=CtrlVcuHevIpsGenTrqMax
  Constant1 : Constant  Value=max(CtrlVcuHevIpsEngTrq)*PlntHevIpsP1SunRingRatio/(1+PlntHevIpsP1SunRingRatio)
  Gain : Gain  Gain=-1
  Saturation Dynamic1 : simulink/Discontinuities/Saturation Dynamic  OutMin=[]  OutMax=[]  OutDataTypeStr=Inherit: Same as second input  OutDataType=fixdt(1, 16)  OutScaling=2^-10  DoSatur=off
  Switch : Switch  Criteria=u2 > Threshold  SaturateOnIntegerOverflow=off  InputSameDT=off
  Out : Outport  VectorParamsAs1DForOutWhenUnconnected=off
  wires:
  Saturation Dynamic1/1 -> Out/1
  Compare To Constant/1 -> Switch/2
  Gain/1 -> Saturation Dynamic1/3
  PI/1 -> Saturation Dynamic1/2
  EngMode/1 -> Compare To Constant/1
  Switch/1 -> Gain/1, Saturation Dynamic1/1
  Constant/1 -> Switch/3
  Constant1/1 -> Switch/1

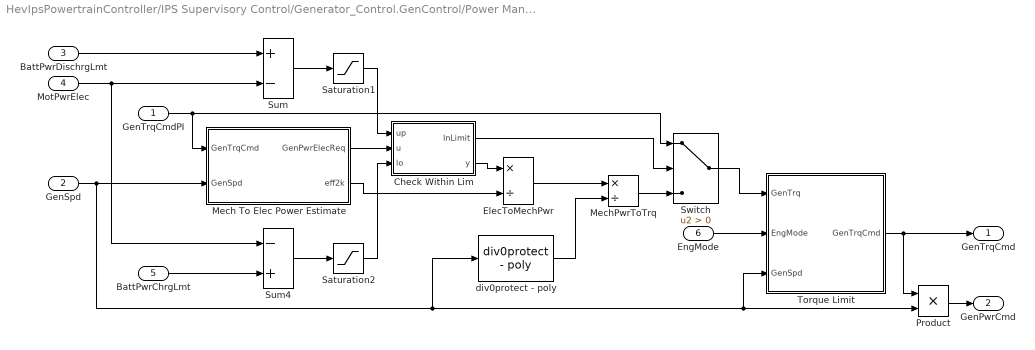
== system HevIpsPowertrainController/IPS Supervisory Control/Generator_Control.GenControl/Power Management ==
  GenTrqCmdPI : Inport
  GenSpd : Inport  Port=2
  BattPwrDischrgLmt : Inport  Port=3
  MotPwrElec : Inport  Port=4
  BattPwrChrgLmt : Inport  Port=5
  EngMode : Inport  Port=6
  Check Within Lim : Subsystem
  ElecToMechPwr : Product  Inputs=*/
  Mech To Elec Power Estimate : Subsystem
  MechPwrToTrq : Product  Inputs=*/
  Product : Product
  Saturation1 : Saturate  UpperLimit=inf  LowerLimit=0
  Saturation2 : Saturate  UpperLimit=0  LowerLimit=-inf
  Sum : Sum  Inputs=+-
  Sum4 : Sum  Inputs=-+
  Switch : Switch  Criteria=u2 > Threshold  SaturateOnIntegerOverflow=off  InputSameDT=off
  Torque Limit : Subsystem
  div0protect - poly : autolibutils/div0protect - poly  thresh=2  ZeroCross1=off  aMode=aMode
  GenTrqCmd : Outport  VectorParamsAs1DForOutWhenUnconnected=off
  GenPwrCmd : Outport  Port=2  VectorParamsAs1DForOutWhenUnconnected=off
  wires:
  BattPwrChrgLmt/1 -> Sum4/2
  Mech To Elec Power Estimate/1(GenPwrElecReq) -> Check Within Lim/2(u)
  Saturation2/1 -> Check Within Lim/3(lo)
  Sum4/1 -> Saturation2/1
  Sum/1 -> Saturation1/1
  Saturation1/1 -> Check Within Lim/1(up)
  MotPwrElec/1 -> Sum/2, Sum4/1
  BattPwrDischrgLmt/1 -> Sum/1
  GenTrqCmdPI/1 -> Mech To Elec Power Estimate/1(GenTrqCmd), Switch/1
  GenSpd/1 -> div0protect - poly/1, Torque Limit/3(GenSpd), Product/2, Mech To Elec Power Estimate/2(GenSpd)
  ElecToMechPwr/1 -> MechPwrToTrq/1
  div0protect - poly/1 -> MechPwrToTrq/2
  Check Within Lim/2(y) -> ElecToMechPwr/1
  Mech To Elec Power Estimate/2(eff2k) -> ElecToMechPwr/2
  Torque Limit/1(GenTrqCmd) -> GenTrqCmd/1, Product/1
  MechPwrToTrq/1 -> Switch/3
  EngMode/1 -> Torque Limit/2(EngMode)
  Product/1 -> GenPwrCmd/1
  Switch/1 -> Torque Limit/1(GenTrq)
  Check Within Lim/1(InLimit) -> Switch/2

== system HevIpsPowertrainController/IPS Supervisory Control/Operating_Modes.Driving.HEV.Low_Power_Charge_Sustain.OpMode3/Torque Blending ==
  note: This function blends the powertrain torque when transitiong from EV mode (using motor)
      | to this Low mode (using engine).  It allows the motor to ramp down it's torque according
      | to the engine torque ramping up.  Once the blending is complete, the motor can begin
      | it's charge sustaining (negative torque) if needed.
  WhlPwrCmd : Inport
  EngTrqOut : Inport  Port=2
  EngSpd : Inport  Port=3
  MotPwrLow : Inport  Port=4
  LPF IC : autolibutils/LPF IC  w=10  aMode=aMode  dataType=off
  Product2 : Product
  Saturation5 : Saturate  UpperLimit=inf  LowerLimit=0
  Sum6 : Sum  Inputs=+-
  Switch : Switch  SaturateOnIntegerOverflow=off  InputSameDT=off
  MotPwrCmd : Outport  VectorParamsAs1DForOutWhenUnconnected=off
  wires:
  MotPwrLow/1 -> Switch/3
  Sum6/1 -> Switch/2, Saturation5/1
  EngTrqOut/1 -> Product2/1
  Saturation5/1 -> Switch/1
  Product2/1 -> Sum6/2  "EngPwrOut"
  EngSpd/1 -> Product2/2
  WhlPwrCmd/1 -> Sum6/1
  Switch/1 -> LPF IC/2, LPF IC/1
  LPF IC/1 -> MotPwrCmd/1

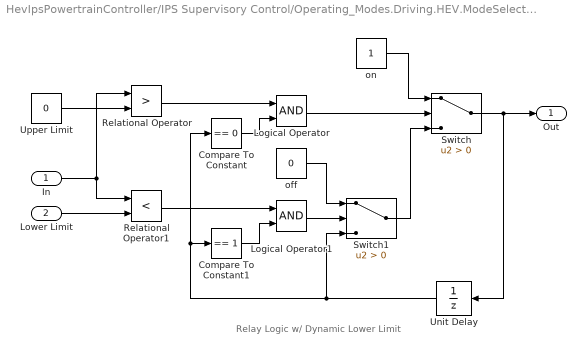
== system HevIpsPowertrainController/IPS Supervisory Control/Operating_Modes.Driving.HEV.ModeSelection/RelayDynLowLimit ==
  note: Relay Logic w/ Dynamic Lower Limit
  In : Inport
  Lower Limit : Inport  Port=2
  Compare To Constant : simulink/Logic and Bit Operations/Compare To Constant  relop===  const=0  OutDataTypeStr=boolean
  Compare To Constant1 : simulink/Logic and Bit Operations/Compare To Constant  relop===  const=1  OutDataTypeStr=boolean
  Logical Operator : Logic  AllPortsSameDT=off  OutDataTypeStr=boolean
  Logical Operator1 : Logic  AllPortsSameDT=off  OutDataTypeStr=boolean
  Relational Operator : RelationalOperator  Operator=>  OutDataTypeStr=boolean  RndMeth=Simplest  InputSameDT=off
  Relational Operator1 : RelationalOperator  Operator=<  OutDataTypeStr=boolean  RndMeth=Simplest  InputSameDT=off
  Switch : Switch  Criteria=u2 > Threshold  SaturateOnIntegerOverflow=off  InputSameDT=off
  Switch1 : Switch  Criteria=u2 > Threshold  SaturateOnIntegerOverflow=off  InputSameDT=off
  Unit Delay : UnitDelay  SampleTime=-1  HasFrameUpgradeWarning=on
  Upper Limit : Constant  Value=0
  off : Constant  Value=0  OutDataTypeStr=boolean
  on : Constant  OutDataTypeStr=boolean
  Out : Outport  VectorParamsAs1DForOutWhenUnconnected=off
  wires:
  In/1 -> Relational Operator1/1, Relational Operator/1
  Upper Limit/1 -> Relational Operator/2
  Lower Limit/1 -> Relational Operator1/2
  Relational Operator/1 -> Logical Operator/1
  Compare To Constant/1 -> Logical Operator/2
  Relational Operator1/1 -> Logical Operator1/1
  Compare To Constant1/1 -> Logical Operator1/2
  Logical Operator/1 -> Switch/2
  on/1 -> Switch/1
  Logical Operator1/1 -> Switch1/2
  off/1 -> Switch1/1
  Switch1/1 -> Switch/3
  Switch/1 -> Unit Delay/1, Out/1
  Unit Delay/1 -> Switch1/3, Compare To Constant/1, Compare To Constant1/1

== system HevIpsPowertrainController/IPS Supervisory Control/Operating_Modes.EngOnCalc/Check Power ==
  note: If Pbatt > PlimBattDischrg
      | for > 0.1 sec, turn EngOn
  BattPwr : Inport
  BattPwrDischrgLmt : Inport  Port=2
  Logical Operator1 : Logic  AllPortsSameDT=off  OutDataTypeStr=boolean
  Relational Operator1 : RelationalOperator  OutDataTypeStr=boolean  RndMeth=Simplest  InputSameDT=off
  Timer : Stateflow chart  TreatAsAtomicUnit=on
  Out : Outport  VectorParamsAs1DForOutWhenUnconnected=off
  wires:
  Logical Operator1/1 -> Out/1
  Timer/1(Out) -> Logical Operator1/2
  BattPwrDischrgLmt/1 -> Relational Operator1/2
  BattPwr/1 -> Relational Operator1/1
  Relational Operator1/1 -> Timer/1(In), Logical Operator1/1

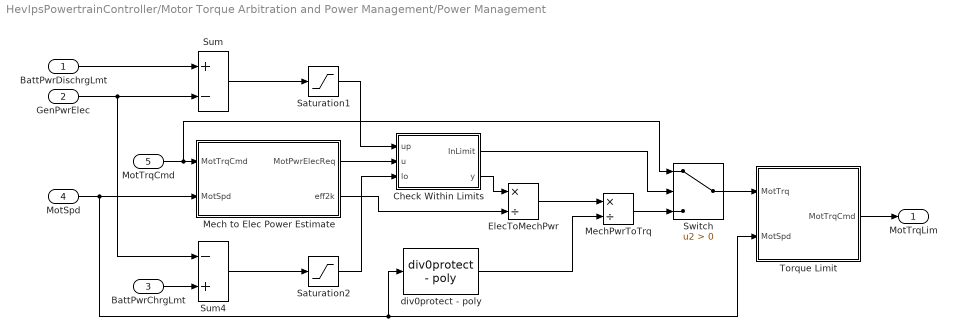
== system HevIpsPowertrainController/Motor Torque Arbitration and Power Management/Power Management ==
  BattPwrDischrgLmt : Inport
  GenPwrElec : Inport  Port=2
  BattPwrChrgLmt : Inport  Port=3
  MotSpd : Inport  Port=4
  MotTrqCmd : Inport  Port=5
  Check Within Limits : Subsystem
  ElecToMechPwr : Product  Inputs=*/
  Mech to Elec Power Estimate : Subsystem
  MechPwrToTrq : Product  Inputs=*/
  Saturation1 : Saturate  UpperLimit=inf  LowerLimit=0
  Saturation2 : Saturate  UpperLimit=0  LowerLimit=-inf
  Sum : Sum  Inputs=+-
  Sum4 : Sum  Inputs=-+
  Switch : Switch  Criteria=u2 > Threshold  SaturateOnIntegerOverflow=off  InputSameDT=off
  Torque Limit : Subsystem
  div0protect - poly : autolibutils/div0protect - poly  thresh=2  ZeroCross1=off  aMode=aMode
  MotTrqLim : Outport  VectorParamsAs1DForOutWhenUnconnected=off
  wires:
  BattPwrChrgLmt/1 -> Sum4/2
  Sum4/1 -> Saturation2/1
  Sum/1 -> Saturation1/1
  GenPwrElec/1 -> Sum/2, Sum4/1
  BattPwrDischrgLmt/1 -> Sum/1
  MotSpd/1 -> Torque Limit/2(MotSpd), div0protect - poly/1, Mech to Elec Power Estimate/2(MotSpd)
  MotTrqCmd/1 -> Switch/1, Mech to Elec Power Estimate/1(MotTrqCmd)
  div0protect - poly/1 -> MechPwrToTrq/2
  Mech to Elec Power Estimate/2(eff2k) -> ElecToMechPwr/2
  ElecToMechPwr/1 -> MechPwrToTrq/1
  MechPwrToTrq/1 -> Switch/3
  Torque Limit/1(MotTrqCmd) -> MotTrqLim/1
  Saturation1/1 -> Check Within Limits/1(up)
  Mech to Elec Power Estimate/1(MotPwrElecReq) -> Check Within Limits/2(u)
  Saturation2/1 -> Check Within Limits/3(lo)
  Check Within Limits/2(y) -> ElecToMechPwr/1
  Switch/1 -> Torque Limit/1(MotTrq)
  Check Within Limits/1(InLimit) -> Switch/2

== system HevIpsPowertrainController/Regen Braking Control/Parallel Regen Braking ==
  VehSpd : Inport
  "MotSpd " : Inport  Port=2
  "BrkPrsReq " : Inport  Port=3
  BattSoc : Inport  Port=4
  ChrgLmt : Lookup_n-D  NumberOfTableDimensions=1  BreakpointsForDimension1=CtrlVcuHevIpsSocBpt  Table=CtrlVcuHevIpsChrgLmtBpt  ExtrapMethod=Clip  UseLastTableValue=on  InternalRulePriority=Speed  RndMeth=Simplest
  Gain : Gain  Gain=-1
  MaxMotTrqVsSpd : Lookup_n-D  NumberOfTableDimensions=1  BreakpointsForDimension1=PlntEM1Spd*30/pi  Table=PlntEM1Trq  ExtrapMethod=Clip  UseLastTableValue=on  InternalRulePriority=Speed  OutDataTypeStr=Inherit: Inherit from 'Table data'  RndMeth=Simplest
  Product1 : Product
  Product3 : Product
  RegenBrakingCutoff : Lookup_n-D  NumberOfTableDimensions=1  BreakpointsForDimension1=CtrlVcuHevIpsRegenBrkSpdBpt  Table=CtrlVcuHevIpsRegenBrkCutOff  ExtrapMethod=Clip  UseLastTableValue=on  InternalRulePriority=Speed  RndMeth=Simplest
  rads_to_rpm : Gain  Gain=30/pi
  " MotTrqCmdRegen" : Outport  VectorParamsAs1DForOutWhenUnconnected=off
  " BrkCmd" : Outport  Port=2  VectorParamsAs1DForOutWhenUnconnected=off
  wires:
  Gain/1 -> " MotTrqCmdRegen"/1  "MotTrqRegen"
  BattSoc/1 -> ChrgLmt/1
  Product3/1 -> Gain/1
  Product1/1 -> Product3/2  "RegenFactor"
  RegenBrakingCutoff/1 -> Product1/1
  VehSpd/1 -> RegenBrakingCutoff/1
  ChrgLmt/1 -> Product1/2
  MaxMotTrqVsSpd/1 -> Product3/1  "MotTrqMax"
  rads_to_rpm/1 -> MaxMotTrqVsSpd/1
  "MotSpd "/1 -> rads_to_rpm/1
  "BrkPrsReq "/1 -> " BrkCmd"/1  "BrkPrsReq"

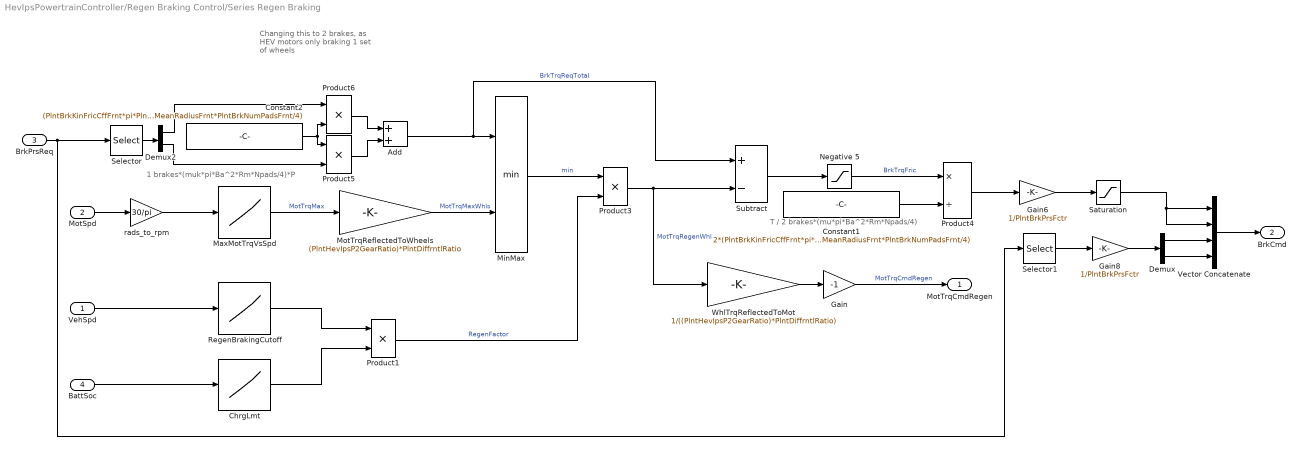
== system HevIpsPowertrainController/Regen Braking Control/Series Regen Braking ==
  note: T / 2 brakes*(mu*pi*Ba^2*Rm*Npads/4)
  note: Changing this to 2 brakes,
      | as HEV motors only braking
      | 1 set of wheels
  note: 1 brakes*(muk*pi*Ba^2*Rm*Npads/4)*P
  VehSpd : Inport
  "MotSpd " : Inport  Port=2
  "BrkPrsReq " : Inport  Port=3
  BattSoc : Inport  Port=4
  Add : Sum
  ChrgLmt : Lookup_n-D  NumberOfTableDimensions=1  BreakpointsForDimension1=CtrlVcuHevIpsSocBpt  Table=CtrlVcuHevIpsChrgLmtBpt  ExtrapMethod=Clip  UseLastTableValue=on  InternalRulePriority=Speed  RndMeth=Simplest
  Constant1 : Constant  Value=2*(PlntBrkKinFricCffFrnt*pi*PlntBrkActrBoreFrnt^2*PlntBrkPadMeanRadiusFrnt*PlntBrkNumPadsFrnt/4)
  Constant2 : Constant  Value=(PlntBrkKinFricCffFrnt*pi*PlntBrkActrBoreFrnt^2*PlntBrkPadMeanRadiusFrnt*PlntBrkNumPadsFrnt/4)
  Demux : Demux  Outputs=2
  Demux2 : Demux  Outputs=2
  Gain : Gain  Gain=-1
  Gain6 : Gain  Gain=1/PlntBrkPrsFctr
  Gain8 : Gain  Gain=1/PlntBrkPrsFctr
  MaxMotTrqVsSpd : Lookup_n-D  NumberOfTableDimensions=1  BreakpointsForDimension1=PlntEM1Spd*30/pi  Table=PlntEM1Trq  ExtrapMethod=Clip  UseLastTableValue=on  InternalRulePriority=Speed  OutDataTypeStr=Inherit: Inherit from 'Table data'  RndMeth=Simplest
  MinMax : MinMax  Inputs=2
  MotTrqReflectedToWheels : Gain  Gain=(PlntHevIpsP2GearRatio)*PlntDiffrntlRatio
  Negative 5 : Saturate  UpperLimit=inf  LowerLimit=0
  Product{1,3,5..6} (4 alike) : Product
  Product4 : Product  Inputs=*/
  RegenBrakingCutoff : Lookup_n-D  NumberOfTableDimensions=1  BreakpointsForDimension1=CtrlVcuHevIpsRegenBrkSpdBpt  Table=CtrlVcuHevIpsRegenBrkCutOff  ExtrapMethod=Clip  UseLastTableValue=on  InternalRulePriority=Speed  RndMeth=Simplest
  Saturation : Saturate  UpperLimit=1  LowerLimit=0
  Selector : Selector  InputPortWidth=4  IndexOptions=Index vector (dialog)  Indices=[1 2]  OutputSizes=1
  Selector1 : Selector  InputPortWidth=4  IndexOptions=Index vector (dialog)  Indices=[3 4]  OutputSizes=1
  Subtract : Sum  Inputs=+-
  Vector Concatenate : Concatenate  NumInputs=4
  WhlTrqReflectedToMot : Gain  Gain=1/((PlntHevIpsP2GearRatio)*PlntDiffrntlRatio)
  rads_to_rpm : Gain  Gain=30/pi
  " MotTrqCmdRegen" : Outport  VectorParamsAs1DForOutWhenUnconnected=off
  " BrkCmd" : Outport  Port=2  VectorParamsAs1DForOutWhenUnconnected=off
  wires:
  Product3/1 -> WhlTrqReflectedToMot/1, Subtract/2  "MotTrqRegenWhl"
  Constant1/1 -> Product4/2
  rads_to_rpm/1 -> MaxMotTrqVsSpd/1
  MaxMotTrqVsSpd/1 -> MotTrqReflectedToWheels/1  "MotTrqMax"
  MinMax/1 -> Product3/1  "min"
  ChrgLmt/1 -> Product1/2
  VehSpd/1 -> RegenBrakingCutoff/1
  RegenBrakingCutoff/1 -> Product1/1
  Product1/1 -> Product3/2  "RegenFactor"
  Subtract/1 -> Negative 5/1
  BattSoc/1 -> ChrgLmt/1
  Negative 5/1 -> Product4/1  "BrkTrqFric"
  "MotSpd "/1 -> rads_to_rpm/1
  MotTrqReflectedToWheels/1 -> MinMax/2  "MotTrqMaxWhls"
  WhlTrqReflectedToMot/1 -> Gain/1
  Gain/1 -> " MotTrqCmdRegen"/1  "MotTrqCmdRegen"
  Add/1 -> MinMax/1, Subtract/1  "BrkTrqReqTotal"
  Selector/1 -> Demux2/1
  Constant2/1 -> Product6/2, Product5/1
  Product6/1 -> Add/1
  Demux2/2 -> Product5/2
  Demux2/1 -> Product6/1
  Product5/1 -> Add/2
  Demux/2 -> Vector Concatenate/4
  Vector Concatenate/1 -> " BrkCmd"/1
  Demux/1 -> Vector Concatenate/3
  Saturation/1 -> Vector Concatenate/2, Vector Concatenate/1
  Gain6/1 -> Saturation/1
  "BrkPrsReq "/1 -> Selector1/1, Selector/1
  Selector1/1 -> Gain8/1
  Product4/1 -> Gain6/1
  Gain8/1 -> Demux/1

== system HevIpsPowertrainController/IPS Supervisory Control/Generator_Control.GenControl/Power Management/Check Within Lim ==
  up : Inport
  u : Inport  Port=2
  lo : Inport  Port=3
  Compare To Zero : simulink/Logic and Bit Operations/Compare To Zero  relop=>=  OutDataTypeStr=boolean
  Compare To Zero1 : simulink/Logic and Bit Operations/Compare To Zero  relop=<=  OutDataTypeStr=boolean
  Logical Operator : Logic  AllPortsSameDT=off  OutDataTypeStr=boolean
  Saturation Dynamic1 : simulink/Discontinuities/Saturation Dynamic  OutMin=[]  OutMax=[]  OutDataTypeStr=Inherit: Same as second input  OutDataType=fixdt(1, 16)  OutScaling=2^-10  DoSatur=off
  Subtract : Sum  Inputs=+-
  Subtract1 : Sum  Inputs=-+
  InLimit : Outport  VectorParamsAs1DForOutWhenUnconnected=off
  y : Outport  Port=2  VectorParamsAs1DForOutWhenUnconnected=off
  wires:
  Saturation Dynamic1/1 -> y/1
  lo/1 -> Subtract1/2, Saturation Dynamic1/3
  up/1 -> Subtract/1, Saturation Dynamic1/1
  u/1 -> Subtract1/1, Subtract/2, Saturation Dynamic1/2
  Subtract/1 -> Compare To Zero/1
  Subtract1/1 -> Compare To Zero1/1
  Compare To Zero/1 -> Logical Operator/1
  Compare To Zero1/1 -> Logical Operator/2
  Logical Operator/1 -> InLimit/1

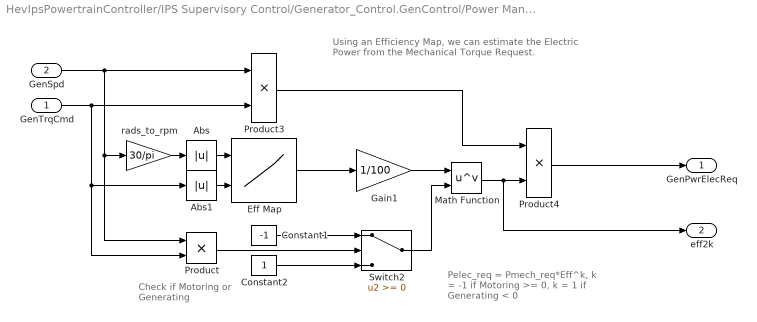
== system HevIpsPowertrainController/IPS Supervisory Control/Generator_Control.GenControl/Power Management/Mech To Elec Power Estimate ==
  note: Check if Motoring
      | or Generating
  note: Using an Efficiency Map, we can estimate the
      | Electric Power from the Mechanical  Torque Request.
  note: Pelec_req = Pmech_req*Eff^k,
      | k = -1 if Motoring >= 0,
      | k = 1 if Generating < 0
  GenTrqCmd : Inport
  GenSpd : Inport  Port=2
  Abs : Abs  SaturateOnIntegerOverflow=off
  Abs1 : Abs  SaturateOnIntegerOverflow=off
  Constant1 : Constant  Value=-1  SampleTime=-1
  Constant2 : Constant  SampleTime=-1
  Eff Map : Lookup_n-D  BreakpointsForDimension1=PlntEM2Spd*30/pi  BreakpointsForDimension2=PlntEM2TrqEff  Table=PlntEM2EffTbl  ExtrapMethod=Clip  UseLastTableValue=on  InternalRulePriority=Speed  OutDataTypeStr=Inherit: Inherit from 'Table data'  RndMeth=Simplest
      settings: InputPortMap=u0,u1
  Gain1 : Gain  Gain=1/100
  Math Function : Math  Operator=pow  SignedPower=on  OutputSignalType=real
  Product : Product
  Product3 : Product
  Product4 : Product
  Switch2 : Switch  SaturateOnIntegerOverflow=off  InputSameDT=off
  rads_to_rpm : Gain  Gain=30/pi
  GenPwrElecReq : Outport  VectorParamsAs1DForOutWhenUnconnected=off
  eff2k : Outport  Port=2  VectorParamsAs1DForOutWhenUnconnected=off
  wires:
  Product3/1 -> Product4/1
  Switch2/1 -> Math Function/2
  Constant1/1 -> Switch2/1
  Constant2/1 -> Switch2/3
  Eff Map/1 -> Gain1/1
  Abs/1 -> Eff Map/1
  Gain1/1 -> Math Function/1
  Math Function/1 -> eff2k/1, Product4/2
  Product4/1 -> GenPwrElecReq/1
  Abs1/1 -> Eff Map/2
  rads_to_rpm/1 -> Abs/1
  Product/1 -> Switch2/2
  GenSpd/1 -> Product3/1, Product/1, rads_to_rpm/1
  GenTrqCmd/1 -> Product3/2, Product/2, Abs1/1

== system HevIpsPowertrainController/IPS Supervisory Control/Generator_Control.GenControl/Power Management/Torque Limit ==
  note: While in Eng Run mode, don't need
      | to have GenTrq > 0, because Gen is
      | braking engine to maintain desired
      | speed.  Using Gen to speed up Eng
      | wastes energy.
  GenTrq : Inport
  EngMode : Inport  Port=2
  GenSpd : Inport  Port=3
  Compare To Constant : simulink/Logic and Bit Operations/Compare To Constant  relop===  const=3  OutDataTypeStr=boolean
  Constant : Constant  Value=0
  Gain : Gain  Gain=-1
  GenMotTrqVsSpd : Lookup_n-D  NumberOfTableDimensions=1  BreakpointsForDimension1=PlntEM2Spd*30/pi  Table=PlntEM2Trq  ExtrapMethod=Clip  UseLastTableValue=on  InternalRulePriority=Speed  OutDataTypeStr=Inherit: Inherit from 'Table data'  RndMeth=Simplest
  Saturation Dynamic : simulink/Discontinuities/Saturation Dynamic  OutMin=[]  OutMax=[]  OutDataTypeStr=Inherit: Same as second input  OutDataType=fixdt(1, 16)  OutScaling=2^-10  DoSatur=off
  Switch : Switch  Criteria=u2 > Threshold  SaturateOnIntegerOverflow=off  InputSameDT=off
  rads_to_rpm : Gain  Gain=30/pi
  GenTrqCmd : Outport  VectorParamsAs1DForOutWhenUnconnected=off
  wires:
  rads_to_rpm/1 -> GenMotTrqVsSpd/1
  Constant/1 -> Switch/1
  GenMotTrqVsSpd/1 -> Switch/3, Gain/1
  Gain/1 -> Saturation Dynamic/3
  GenTrq/1 -> Saturation Dynamic/2
  Saturation Dynamic/1 -> GenTrqCmd/1
  GenSpd/1 -> rads_to_rpm/1
  EngMode/1 -> Compare To Constant/1
  Compare To Constant/1 -> Switch/2
  Switch/1 -> Saturation Dynamic/1

== system HevIpsPowertrainController/Motor Torque Arbitration and Power Management/Power Management/Check Within Limits ==
  up : Inport
  u : Inport  Port=2
  lo : Inport  Port=3
  Compare To Zero : simulink/Logic and Bit Operations/Compare To Zero  relop=>=  OutDataTypeStr=boolean
  Compare To Zero1 : simulink/Logic and Bit Operations/Compare To Zero  relop=<=  OutDataTypeStr=boolean
  Logical Operator : Logic  AllPortsSameDT=off  OutDataTypeStr=boolean
  Saturation Dynamic1 : simulink/Discontinuities/Saturation Dynamic  OutMin=[]  OutMax=[]  OutDataTypeStr=Inherit: Same as second input  OutDataType=fixdt(1, 16)  OutScaling=2^-10  DoSatur=off
  Subtract : Sum  Inputs=+-
  Subtract1 : Sum  Inputs=-+
  InLimit : Outport  VectorParamsAs1DForOutWhenUnconnected=off
  y : Outport  Port=2  VectorParamsAs1DForOutWhenUnconnected=off
  wires:
  Saturation Dynamic1/1 -> y/1
  lo/1 -> Subtract1/2, Saturation Dynamic1/3
  up/1 -> Subtract/1, Saturation Dynamic1/1
  u/1 -> Subtract1/1, Subtract/2, Saturation Dynamic1/2
  Subtract/1 -> Compare To Zero/1
  Subtract1/1 -> Compare To Zero1/1
  Compare To Zero/1 -> Logical Operator/1
  Compare To Zero1/1 -> Logical Operator/2
  Logical Operator/1 -> InLimit/1
